simulink library "NCS_Library"  (R2019a)
settings: Solver=VariableStepAuto  StartTime=0.0  StopTime=10.0  RelTol=1e-3
values from neighbouring files (symbols this model uses):
  A = 10    [Parameter.m]
  band = 100000000    [Parameter.m]
  BER = 0    [Parameter.m]
  c = 5000000    [Parameter.m]
  c1 = 4.33    [Parameter.m]
  c2 = 3.16    [Parameter.m]
  CAN2EthernetDelay = 0.000    (= 0)    [Parameter.m]
  cR = 1.5*10^-3    (= 0.0015)    [Parameter.m]
  cw = (cwE * 2 + cwM * (nW_ges-2))/nW_ges    (= 0.1475)    [Parameter.m]
  cwE = 0.35    [Parameter.m]
  cwM = 0.08    [Parameter.m]
  Cycle_Controller = 0    [Parameter.m]
  CyclePLC = 24/1000    (= 0.024)    [Parameter.m]
  d = 800000    [Parameter.m]
  Dr = 0.92    [Parameter.m]
  Ethernet2CANDelay = 0.005    [Parameter.m]
  F_konst = 70892    [Parameter.m]
  FA = 100000    [Parameter.m]
  FB_WB_max = 10000    [Parameter.m]
  FBel_an = iG*nG*F_KZmax*nBan*R_mR/(Dr/2)    (= 28197.4297239)    [Parameter.m]
  FBel_frei = iG*nG*F_KZmax*nBfrei*R_mW/(Dr/2)    (= 29270.6882948)    [Parameter.m]
  Fmaxdyn = 300000    [Parameter.m]
  g = 9.81    [Parameter.m]
  i = 0    [Parameter.m]
  J = 1/2*mA*(Dr/2)^2    (= 158.7)    [Parameter.m]
  k1 = 0.095    [Parameter.m]
  k2 = 9.26/3.6    (= 2.57222222222)    [Parameter.m]
  k3 = 4.63/3.6    (= 1.28611111111)    [Parameter.m]
  mges = 58000    [Parameter.m]
  mu = [mu1 mu2]    [Parameter.m]
  muBel1 = 0.42    [Parameter.m]
  muBel2 = 0.36    [Parameter.m]
  n = 0.001    [Parameter.m]
  n_Mg = 4    [Parameter.m]
  n_WB = 4    [Parameter.m]
  nA = 4    [Parameter.m]
  nBan = 2    [Parameter.m]
  nBfrei = 3    [Parameter.m]
  nM = 4    [Parameter.m]
  nW_an = 4    [Parameter.m]
  P_max = 8200000    [Parameter.m]
  Q = 10    [Parameter.m]
  r_reib = 600    [Parameter.m]
  rho = 1.08    [Parameter.m]
  rhoL = 1.225    [Parameter.m]
  Size = 8    [Parameter.m]
  slip = [s1 s2]    [Parameter.m]
  tol = 0.05    [Parameter.m]
  v00 = 100/3.6    (= 27.7777777778)    [Parameter.m]
  v_grenz = 60/3.6    (= 16.6666666667)    [Parameter.m]
  v_opt = 75/3.6    (= 20.8333333333)    [Parameter.m]
  W_opt = 0.5    [Parameter.m]
  WB = 1    [Parameter.m]
  y_opt = sqrt(W_opt)/((1+sqrt(W_opt))^2+W_opt)    [Parameter.m]
undefined symbols (not defined in the file or in its folder): BUSCapacity, CableLength, controlGate, D_dyn, D_mg, EnableBurst, EnableToF, entity, Entity_out, Gate, Gate_4, Gate_5, Gate_ACK, Gate_copy, Gate_RX, getData, gettime, I_dyn, I_mg, m, magnitude, P_dyn, P_mg, ReadAttributes, readdata, ReadData, ReadSize, sigbuilder_block, Timeout, ToB, ToF, v0, v_d, v_soll
libraries: simulink x176, $bdroot x102
(part 4 of 12)

== system NCS_Library/Network/ETB/Controller Interface ==
  Rx : Inport
  U : Inport  Port=2
  Clock : Clock
  Compare To Constant : simulink/Logic and Bit Operations/Compare To Constant  relop=>=  const=ToF  OutDataTypeStr=uint8
  Constant : Constant  Value=EnableToF
  Data Type Conversion : DataTypeConversion  OutDataTypeStr=uint8
  Display1 : Display
  Display2 : Display
  Failure Control : $bdroot/Network/Applications/Failure Control  SystemSampleTime=-1
  Failure Control1 : $bdroot/Network/Applications/Failure Control  SystemSampleTime=-1
  Logical Operator : Logic  AllPortsSameDT=off  OutDataTypeStr=boolean
  Parameter : Subsystem
  Subsystem : Subsystem
  Tx : Outport
  Recorder : Outport  Port=2
  Failed : Outport  Port=3
  Y_M : Outport  Port=4
  wires:
  Rx/1 -> Failure Control1/1
  Subsystem/3(TxToBus) -> Failure Control/1
  U/1 -> Subsystem/1(InFromController)
  Subsystem/1(OutToController) -> Y_M/1
  Failure Control1/1 -> Subsystem/3(RxFromBus)
  Parameter/1(Out1) -> Subsystem/2(Parameter)
  Failure Control/1 -> Tx/1
  Compare To Constant/1 -> Logical Operator/1, Display1/1
  Logical Operator/1 -> Data Type Conversion/1, Display2/1
  Clock/1 -> Compare To Constant/1
  Constant/1 -> Logical Operator/2
  Data Type Conversion/1 -> Failed/1
  Subsystem/2(Recorder) -> Recorder/1

== system NCS_Library/Network/ETB/ED ==
  RxFromBus : Inport
  Signal : Inport  Port=2
  Failure Control Rx : $bdroot/Network/Applications/Failure Control  SystemSampleTime=-1
  Failure Control Tx : $bdroot/Network/Applications/Failure Control  SystemSampleTime=-1
  Protocol Stack : Subsystem
  User Interface : Subsystem
  TxToBus : Outport
  Recorder : Outport  Port=2
  ReceivedData : Outport  Port=3
  wires:
  Protocol Stack/2(Recorder) -> Recorder/1
  Protocol Stack/1(Data) -> ReceivedData/1
  Signal/1 -> Protocol Stack/1(Signal)
  RxFromBus/1 -> Failure Control Rx/1
  Protocol Stack/3(TxToBus) -> Failure Control Tx/1
  Failure Control Rx/1 -> Protocol Stack/3(RxFromBus)
  Failure Control Tx/1 -> TxToBus/1
  User Interface/1(Parameter) -> Protocol Stack/2(Parameter)

== system NCS_Library/Network/ETB/Ethernet_2-port_Switch ==
  note: Address_Memory
  from_S : Inport
  from_N : Inport  Port=2
  Address_Storage Poer_S : DataStoreMemory  DataStoreName=S  ReadBeforeWriteMsg=warning  WriteAfterWriteMsg=warning  WriteAfterReadMsg=warning  InitialValue=zeros(1, addstore)  ShowAdditionalParam=off
  Address_Storage Port_N : DataStoreMemory  DataStoreName=N  ReadBeforeWriteMsg=warning  WriteAfterWriteMsg=warning  WriteAfterReadMsg=warning  InitialValue=zeros(1, addstore)  ShowAdditionalParam=off
  Buffer_Full_ Frame_loss1 : EntityTerminator  InputPortMessageModes=m  NumberEntitiesArrived=on
      settings: OutputPortMap=o0
  Buffer_Full_Frame_loss : EntityTerminator  InputPortMessageModes=m  NumberEntitiesArrived=on
      settings: OutputPortMap=o0
  Buffer_fill Control : Subsystem
  Buffer_fill Control1 : Subsystem
  Determine Port_L/R : Subsystem  TreatAsAtomicUnit=on
  Determine Port_N : Subsystem  TreatAsAtomicUnit=on
  Display{,1..3} (4 alike) : Display
  Entity Input Switch : EntityInputSwitch  InputPortMessageModes=m,m  OutputPortMessageModes=m
  Entity Input Switch1 : EntityInputSwitch  InputPortMessageModes=m,m  OutputPortMessageModes=m
  Entity Output Switch : EntityOutputSwitch  InputPortMessageModes=m  OutputPortMessageModes=m,m,m  NumberOutputPorts=3  SwitchingCriterion=From attribute  SwitchAttributeName=Route
      settings: OutputPortMap=o0,o1,o2
  Entity Output Switch1 : EntityOutputSwitch  InputPortMessageModes=m,m  OutputPortMessageModes=m,m  SwitchingCriterion=From control port  SwitchAttributeName=Attribute1
      settings: InputPortMap=u0,u1
  Entity Output Switch2 : EntityOutputSwitch  InputPortMessageModes=m  OutputPortMessageModes=m,m,m  NumberOutputPorts=3  SwitchingCriterion=From attribute  SwitchAttributeName=Route
      settings: OutputPortMap=o0,o1,o2
  Entity Output Switch3 : EntityOutputSwitch  InputPortMessageModes=m,m  OutputPortMessageModes=m,m  SwitchingCriterion=From control port  SwitchAttributeName=Attribute1
      settings: InputPortMap=u0,u1
  Entity Queue : EntityQueue  InputPortMessageModes=m  OutputPortMessageModes=m
      settings: OutputPortMap=o5
  Entity Queue1 : EntityQueue  InputPortMessageModes=m  OutputPortMessageModes=m
      settings: OutputPortMap=o5
  Entity Replicator : EntityReplicator  InputPortMessageModes=m  OutputPortMessageModes=m,m
  Entity Terminator : EntityTerminator  InputPortMessageModes=m
  Not_for_ here_Terminate : EntityTerminator  InputPortMessageModes=m
  Output Buffer N : EntityQueue  InputPortMessageModes=m  OutputPortMessageModes=n,m  Capacity=floor(buffer_size/(2*1500))  NumberEntitiesInBlock=on
      settings: OutputPortMap=o1,o5
  Output Buffer R/L : EntityQueue  InputPortMessageModes=m  OutputPortMessageModes=n,m  Capacity=floor(buffer_size/(2*1500))  NumberEntitiesInBlock=on
      settings: OutputPortMap=o1,o5
  Output_Time_N : EntityServer  InputPortMessageModes=m  OutputPortMessageModes=n,m  Capacity=1  ServiceTimeSource=Attribute  NumberEntitiesDeparted=on
      settings: OutputPortMap=o0,o9
  Output_Time_R/L : EntityServer  InputPortMessageModes=m  OutputPortMessageModes=n,m  Capacity=1  ServiceTimeSource=Attribute  NumberEntitiesDeparted=on
      settings: OutputPortMap=o0,o9
  Swicth_Logic_R/L : EntityServer  InputPortMessageModes=m  OutputPortMessageModes=m  Capacity=1  ServiceTimeValue=CycleSwitch  EntryAction=[entity.Route, entity.ServiceTime] = gate_s(entity.MACDestination, entity.MACSource, entity.Size);
  Switch_Logic_N : EntityServer  InputPortMessageModes=m  OutputPortMessageModes=m  Capacity=1  ServiceTimeValue=CycleSwitch  EntryAction=[entity.Route, entity.ServiceTime] = gate_n(entity.MACDestination, entity.MACSource, entity.Size);
  Terminate_ broadcast_ frame : EntityTerminator  InputPortMessageModes=m
  to_S : Outport
  to_N : Outport  Port=2
  wires:
  Buffer_Full_Frame_loss/1 -> Display1/1
  Buffer_Full_ Frame_loss1/1 -> Display/1
  Output Buffer N/2 -> Output_Time_N/1
  Entity Output Switch3/1 -> Output Buffer N/1
  Output Buffer N/1 -> Buffer_fill Control1/1(In1)
  Buffer_fill Control1/1(Out1) -> Entity Output Switch3/1
  Entity Output Switch3/2 -> Buffer_Full_ Frame_loss1/1
  Output Buffer R/L/2 -> Output_Time_R/L/1
  Entity Output Switch1/1 -> Output Buffer R/L/1
  Output Buffer R/L/1 -> Buffer_fill Control/1(In1)
  Buffer_fill Control/1(Out1) -> Entity Output Switch1/1
  Entity Output Switch1/2 -> Buffer_Full_Frame_loss/1
  from_N/1 -> Entity Queue/1
  Switch_Logic_N/1 -> Entity Output Switch/1
  Output_Time_N/2 -> to_N/1
  from_S/1 -> Entity Queue1/1
  Output_Time_R/L/2 -> to_S/1
  Swicth_Logic_R/L/1 -> Entity Output Switch2/1
  Entity Input Switch/1 -> Entity Output Switch3/2
  Entity Output Switch2/2 -> Entity Input Switch/1
  Entity Output Switch/1 -> Entity Terminator/1
  Entity Output Switch/2 -> Entity Input Switch1/1
  Entity Output Switch/3 -> Entity Input Switch1/2
  Entity Input Switch1/1 -> Entity Output Switch1/2
  Entity Output Switch2/3 -> Entity Replicator/1
  Entity Output Switch2/1 -> Not_for_ here_Terminate/1
  Entity Replicator/1 -> Entity Input Switch/2
  Entity Replicator/2 -> Terminate_ broadcast_ frame/1
  Output_Time_R/L/1 -> Display2/1
  Output_Time_N/1 -> Display3/1
  Entity Queue1/1 -> Swicth_Logic_R/L/1
  Entity Queue/1 -> Switch_Logic_N/1

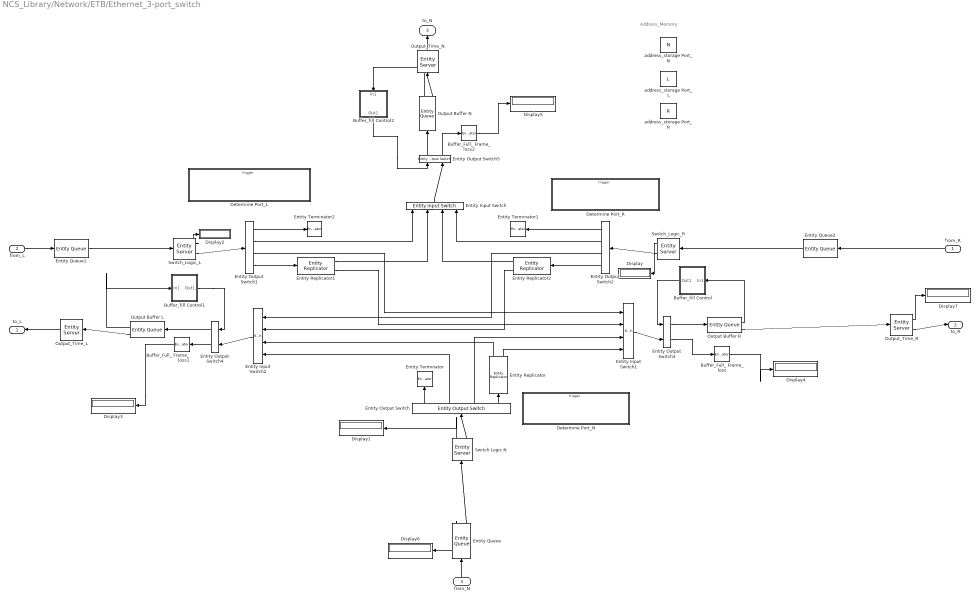
== system NCS_Library/Network/ETB/Ethernet_3-port_switch ==
  note: Address_Memory
  from_R : Inport
  from_L : Inport  Port=2
  from_N : Inport  Port=3
  Buffer_Full_ Frame_loss : EntityTerminator  InputPortMessageModes=m  NumberEntitiesArrived=on
      settings: OutputPortMap=o0
  Buffer_Full_ Frame_loss1 : EntityTerminator  InputPortMessageModes=m  NumberEntitiesArrived=on
      settings: OutputPortMap=o0
  Buffer_Full_ Frame_loss2 : EntityTerminator  InputPortMessageModes=m  NumberEntitiesArrived=on
      settings: OutputPortMap=o0
  Buffer_fill Control : Subsystem
  Buffer_fill Control1 : Subsystem
  Buffer_fill Control2 : Subsystem
  Determine Port_L : Subsystem  TreatAsAtomicUnit=on
  Determine Port_N : Subsystem  TreatAsAtomicUnit=on
  Determine Port_R : Subsystem  TreatAsAtomicUnit=on
  Display{,1..7} (8 alike) : Display
  Entity Input Switch : EntityInputSwitch  InputPortMessageModes=m,m,m,m  OutputPortMessageModes=m  NumberInputPorts=4
      settings: InputPortMap=u1,u2,u3,u4
  Entity Input Switch1 : EntityInputSwitch  InputPortMessageModes=m,m,m,m  OutputPortMessageModes=m  NumberInputPorts=4
      settings: InputPortMap=u1,u2,u3,u4
  Entity Input Switch2 : EntityInputSwitch  InputPortMessageModes=m,m,m,m  OutputPortMessageModes=m  NumberInputPorts=4
      settings: InputPortMap=u1,u2,u3,u4
  Entity Output Switch : EntityOutputSwitch  InputPortMessageModes=m  OutputPortMessageModes=m,m,m,m  NumberOutputPorts=4  SwitchingCriterion=From attribute  SwitchAttributeName=Route
      settings: OutputPortMap=o0,o1,o2,o3
  Entity Output Switch1 : EntityOutputSwitch  InputPortMessageModes=m  OutputPortMessageModes=m,m,m,m  NumberOutputPorts=4  SwitchingCriterion=From attribute  SwitchAttributeName=Route
      settings: OutputPortMap=o0,o1,o2,o3
  Entity Output Switch2 : EntityOutputSwitch  InputPortMessageModes=m  OutputPortMessageModes=m,m,m,m  NumberOutputPorts=4  SwitchingCriterion=From attribute  SwitchAttributeName=Route
      settings: OutputPortMap=o0,o1,o2,o3
  Entity Output Switch3 : EntityOutputSwitch  InputPortMessageModes=m,m  OutputPortMessageModes=m,m  SwitchingCriterion=From control port  SwitchAttributeName=Attribute1
      settings: InputPortMap=u0,u1
  Entity Output Switch4 : EntityOutputSwitch  InputPortMessageModes=m,m  OutputPortMessageModes=m,m  SwitchingCriterion=From control port  SwitchAttributeName=Attribute1
      settings: InputPortMap=u0,u1
  Entity Output Switch5 : EntityOutputSwitch  InputPortMessageModes=m,m  OutputPortMessageModes=m,m  SwitchingCriterion=From control port  SwitchAttributeName=Attribute1
      settings: InputPortMap=u0,u1
  Entity Queue : EntityQueue  InputPortMessageModes=m  OutputPortMessageModes=n,m  NumberEntitiesInBlock=on
      settings: OutputPortMap=o1,o5
  Entity Queue1 : EntityQueue  InputPortMessageModes=m  OutputPortMessageModes=m
      settings: OutputPortMap=o5
  Entity Queue2 : EntityQueue  InputPortMessageModes=m  OutputPortMessageModes=m
      settings: OutputPortMap=o5
  Entity Replicator : EntityReplicator  InputPortMessageModes=m  OutputPortMessageModes=m,m
  Entity Replicator1 : EntityReplicator  InputPortMessageModes=m  OutputPortMessageModes=m,m
  Entity Replicator2 : EntityReplicator  InputPortMessageModes=m  OutputPortMessageModes=m,m
  Entity Terminator : EntityTerminator  InputPortMessageModes=m
  Entity Terminator1 : EntityTerminator  InputPortMessageModes=m
  Entity Terminator2 : EntityTerminator  InputPortMessageModes=m
  Output Buffer L : EntityQueue  InputPortMessageModes=m  OutputPortMessageModes=n,m  Capacity=floor(buffer_size/(3*1500))  NumberEntitiesInBlock=on
      settings: OutputPortMap=o1,o5
  Output Buffer N : EntityQueue  InputPortMessageModes=m  OutputPortMessageModes=n,m  Capacity=floor(buffer_size/(3*1500))  NumberEntitiesInBlock=on
      settings: OutputPortMap=o1,o5
  Output Buffer R : EntityQueue  InputPortMessageModes=m  OutputPortMessageModes=n,m  Capacity=floor(buffer_size/(3*1500))  NumberEntitiesInBlock=on
      settings: OutputPortMap=o1,o5
  Output_Time_L : EntityServer  InputPortMessageModes=m  OutputPortMessageModes=m  Capacity=1  ServiceTimeSource=Attribute
  Output_Time_N : EntityServer  InputPortMessageModes=m  OutputPortMessageModes=m  Capacity=1  ServiceTimeSource=Attribute
  Output_Time_R : EntityServer  InputPortMessageModes=m  OutputPortMessageModes=n,m  Capacity=1  ServiceTimeSource=Attribute  AverageWait=on
      settings: OutputPortMap=o4,o9
  Switch Logic N : EntityServer  InputPortMessageModes=m  OutputPortMessageModes=n,m  Capacity=1  ServiceTimeValue=CycleSwitch  EntryAction=[entity.Route, entity.ServiceTime] = gate_n(entity.MACDestination, entity.MACSource, entity.Size);  NumberEntitiesDeparted=on
      settings: OutputPortMap=o0,o9
  Switch_Logic_L : EntityServer  InputPortMessageModes=m  OutputPortMessageModes=n,m  Capacity=1  ServiceTimeValue=CycleSwitch  EntryAction=[entity.Route, entity.ServiceTime] = gate_l(entity.MACDestination, entity.MACSource, entity.Size);  NumberEntitiesDeparted=on
      settings: OutputPortMap=o0,o9
  Switch_Logic_R : EntityServer  InputPortMessageModes=m  OutputPortMessageModes=n,m  Capacity=1  ServiceTimeValue=CycleSwitch  EntryAction=[entity.Route, entity.ServiceTime] = gate_r(entity.MACDestination, entity.MACSource, entity.Size);  NumberEntitiesDeparted=on
      settings: OutputPortMap=o0,o9
  address_storage Port_L : DataStoreMemory  DataStoreName=L  InitialValue=zeros(1, addstore)  ShowAdditionalParam=off
  address_storage Port_N : DataStoreMemory  DataStoreName=N  InitialValue=zeros(1, addstore)  ShowAdditionalParam=off
  address_storage Port_R : DataStoreMemory  DataStoreName=R  ReadBeforeWriteMsg=warning  WriteAfterWriteMsg=warning  WriteAfterReadMsg=warning  InitialValue=zeros(1, addstore)  ShowAdditionalParam=off
  to_L : Outport
  to_R : Outport  Port=2
  to_N : Outport  Port=3
  wires:
  from_N/1 -> Entity Queue/1
  Switch Logic N/2 -> Entity Output Switch/1
  from_L/1 -> Entity Queue1/1
  Switch_Logic_L/2 -> Entity Output Switch1/1
  Switch_Logic_R/2 -> Entity Output Switch2/1
  from_R/1 -> Entity Queue2/1
  Switch Logic N/1 -> Display1/1
  Output_Time_R/2 -> to_R/1
  Entity Input Switch2/1 -> Entity Output Switch4/2
  Output_Time_L/1 -> to_L/1
  Switch_Logic_L/1 -> Display2/1
  Switch_Logic_R/1 -> Display/1
  Output_Time_R/1 -> Display7/1
  Output Buffer R/2 -> Output_Time_R/1
  Entity Output Switch3/2 -> Buffer_Full_ Frame_loss/1
  Buffer_fill Control/1(Out1) -> Entity Output Switch3/1
  Output Buffer R/1 -> Buffer_fill Control/1(In1)
  Entity Output Switch3/1 -> Output Buffer R/1
  Entity Input Switch1/1 -> Entity Output Switch3/2
  Entity Replicator2/2 -> Entity Input Switch2/2
  Entity Output Switch2/3 -> Entity Input Switch2/1
  Entity Output Switch4/1 -> Output Buffer L/1
  Output Buffer L/1 -> Buffer_fill Control1/1(In1)
  Entity Output Switch4/2 -> Buffer_Full_ Frame_loss1/1
  Buffer_fill Control1/1(Out1) -> Entity Output Switch4/1
  Output Buffer L/2 -> Output_Time_L/1
  Entity Replicator1/2 -> Entity Input Switch1/2
  Entity Output Switch1/2 -> Entity Input Switch/1
  Output_Time_N/1 -> to_N/1
  Entity Output Switch5/1 -> Output Buffer N/1
  Entity Input Switch/1 -> Entity Output Switch5/2
  Output Buffer N/1 -> Buffer_fill Control2/1(In1)
  Entity Output Switch5/2 -> Buffer_Full_ Frame_loss2/1
  Buffer_fill Control2/1(Out1) -> Entity Output Switch5/1
  Output Buffer N/2 -> Output_Time_N/1
  Buffer_Full_ Frame_loss1/1 -> Display3/1
  Buffer_Full_ Frame_loss2/1 -> Display5/1
  Buffer_Full_ Frame_loss/1 -> Display4/1
  Entity Output Switch/1 -> Entity Terminator/1
  Entity Output Switch/2 -> Entity Input Switch2/4
  Entity Output Switch/3 -> Entity Input Switch1/3
  Entity Output Switch/4 -> Entity Replicator/1
  Entity Replicator/2 -> Entity Input Switch1/4
  Entity Replicator/1 -> Entity Input Switch2/3
  Entity Output Switch2/4 -> Entity Replicator2/1
  Entity Output Switch2/1 -> Entity Terminator1/1
  Entity Output Switch2/2 -> Entity Input Switch/4
  Entity Replicator2/1 -> Entity Input Switch/3
  Entity Output Switch1/4 -> Entity Replicator1/1
  Entity Replicator1/1 -> Entity Input Switch/2
  Entity Output Switch1/3 -> Entity Input Switch1/1
  Entity Output Switch1/1 -> Entity Terminator2/1
  Entity Queue2/1 -> Switch_Logic_R/1
  Entity Queue/2 -> Switch Logic N/1
  Entity Queue1/1 -> Switch_Logic_L/1
  Entity Queue/1 -> Display6/1

== system NCS_Library/Network/ETB/OSI Layers ==
  note: Application
  note: Layer 6
  note: Layer 5
  note: Layer 4
  note: Layer 3
  note: Layer 1&2
  Application : Subsystem  mask{Port=1}
      mask Display: disp('App')
  IP : Subsystem
  MAC Controller : Subsystem
  SDTv2 : Subsystem
  TRDP PD : Subsystem
  TRDP Timeout : Subsystem
  UDP Multi-Port : Subsystem
  UDP Single-Port : Subsystem

== system NCS_Library/Network/ETB/Subsystem2 ==
  InSubnet1 : Inport
  InSubnet2 : Inport  Port=2
  InSubnet3 : Inport  Port=3
  MAC Layer : Subsystem
  Routing Layer : Subsystem
  Routing Table : Subsystem
  User Interface : Subsystem
  OutSubnet1 : Outport
  OutSubnet2 : Outport  Port=2
  OutSubnet3 : Outport  Port=3
  wires:
  MAC Layer/3(OutToIP3) -> Routing Layer/4(InSubnet3)
  Routing Layer/1(OutSubnet3) -> MAC Layer/3(InFromIP3)
  MAC Layer/6(OutToSubnet3) -> OutSubnet3/1
  InSubnet3/1 -> MAC Layer/7(InFromSubnet3)
  Routing Table/1(RT) -> Routing Layer/2(Routing Table)
  MAC Layer/5(OutSubnet2) -> OutSubnet2/1
  MAC Layer/4(OutToSubnet1) -> OutSubnet1/1
  InSubnet2/1 -> MAC Layer/6(InFromSubnet2)
  InSubnet1/1 -> MAC Layer/5(InFromSubnet1)
  MAC Layer/2(OutToIP2) -> Routing Layer/5(InSubnet2)
  MAC Layer/1(OutIP1) -> Routing Layer/6(InSubnet1)
  Routing Layer/2(OutSubnet2) -> MAC Layer/2(InFromIP2)
  Routing Layer/3(OutSubnet1) -> MAC Layer/1(InIP1)
  Routing Table/2(FIN) -> Routing Layer/1(FIN)
  User Interface/1(Paramter) -> Routing Table/1(Parameter), Routing Layer/3(Parameter), MAC Layer/4(Parameter)

== system NCS_Library/Network/ETB/Termination ==
  IN : Inport
  Display : Display
  Entity Generator1 : EntityGenerator  InputPortMessageModes=m  OutputPortMessageModes=m  GenerationMethod=Event-based  TimeSource=Signal port  GenerateEntityAtSimulationStart=off  EntityType=Bus object  EntityTypeName=Ethernet_Entity
      settings: InputPortMap=u0
  Entity Terminator : EntityTerminator  InputPortMessageModes=m  NumberEntitiesArrived=on
      settings: OutputPortMap=o0
  Ground1 : Ground
  OUT : Outport
  wires:
  IN/1 -> Entity Terminator/1
  Entity Terminator/1 -> Display/1
  Entity Generator1/1 -> OUT/1
  Ground1/1 -> Entity Generator1/1

== system NCS_Library/Network/Gateway/Gateway1 ==
  In1 : Inport
  CAN Interface : Subsystem
  Ethernet Interface : Subsystem
  Out1 : Outport
  wires:
  CAN Interface/1(OutEthernetData) -> Ethernet Interface/2(CANData)
  Ethernet Interface/2(ReceivedData) -> CAN Interface/1(ReceivedData)
  In1/1 -> Ethernet Interface/1(RxFromBus)
  Ethernet Interface/1(TxToBus) -> Out1/1

== system NCS_Library/Network/Gateway/Gateway2 ==
  In1 : Inport
  CAN Interface : Subsystem
  Ethernet Interface : Subsystem
  Out1 : Outport
  wires:
  Ethernet Interface/1(TxToBus) -> Out1/1
  In1/1 -> Ethernet Interface/1(RxFromBus)
  Ethernet Interface/2(ReceivedData) -> CAN Interface/1(ReceivedData)
  CAN Interface/1(OutEthernetData) -> Ethernet Interface/2(CANData)

== system NCS_Library/Plant (Train)/Angetriebene_Achse/Bremskraft pro angetriebener Achse2 ==
  v : Inport
  f_St,dyn : Inport  Port=2
  f_St_pneumatic : Inport  Port=3
  Add : Sum
  Belagreibwert_Nennwerte : Subsystem
  Belagskraft pro Achse : Constant  Value=FBel_an
  Compare To Constant3 : simulink/Logic and Bit Operations/Compare To Constant  relop=>=  const=0  OutDataTypeStr=boolean
  Display : Display
  Display1 : Display
  Display2 : Display
  Product : Product  Inputs=3
  Product1 : Product  Inputs=3
  Switch : Switch  Criteria=u2 > Threshold
  f_St,dyn1 : InportShadow  Port=2
  max dynamische Bremse pro angetriebener Achse1 : Subsystem
  max dynamische Motor pro angetriebener Achse : Subsystem
  F_B,A : Outport
  wires:
  Belagreibwert_Nennwerte/1(mu_Bel) -> Product/1
  Belagskraft pro Achse/1 -> Product/2
  f_St_pneumatic/1 -> Product/3  "f_St_pneumatic"
  v/1 -> Belagreibwert_Nennwerte/1(v), max dynamische Motor pro angetriebener Achse/1(v), max dynamische Bremse pro angetriebener Achse1/1(v), Compare To Constant3/1
  Product/1 -> Display1/1, Add/2
  Add/1 -> Display2/1, F_B,A/1
  Product1/1 -> Display/1, Add/1
  max dynamische Motor pro angetriebener Achse/1(F_B,dyn_max) -> Switch/3
  Compare To Constant3/1 -> Product1/3
  f_St,dyn/1 -> Product1/1
  max dynamische Bremse pro angetriebener Achse1/1(F_B,dyn_max) -> Switch/1
  f_St,dyn1/1 -> Switch/2
  Switch/1 -> Product1/2

== system NCS_Library/Plant (Train)/Freie_Achse/Bremskraft pro freier Achse1 ==
  v : Inport
  fSt Achse 1 : Inport  Port=2
  Belagreibwert_Nennwerte : Subsystem
  Belagskraft : Constant  Value=FBel_frei
  Display : Display
  Product : Product  Inputs=3
  F_B : Outport
  wires:
  Product/1 -> F_B/1
  Belagreibwert_Nennwerte/1(muBel) -> Product/1
  v/1 -> Belagreibwert_Nennwerte/1(v)
  fSt Achse 1/1 -> Display/1, Product/3
  Belagskraft/1 -> Product/2

== system NCS_Library/Plant (Train)/Kupplung/Dämpferkraft1-2 ==
  v1 : Inport
  v2 : Inport  Port=2
  Add : Sum  Inputs=+-
  Dämpferkonstante : Gain  Gain=d
  Fd1-2 : Outport
  wires:
  Dämpferkonstante/1 -> Fd1-2/1
  Add/1 -> Dämpferkonstante/1
  v2/1 -> Add/2
  v1/1 -> Add/1

== system NCS_Library/Plant (Train)/Kupplung/Federkraft1-2 ==
  s1 : Inport
  s2 : Inport  Port=2
  Add : Sum  Inputs=+-
  Federkonstante : Gain  Gain=c
  Ff1-2 : Outport
  wires:
  Federkonstante/1 -> Ff1-2/1
  Add/1 -> Federkonstante/1
  s2/1 -> Add/2
  s1/1 -> Add/1

== system NCS_Library/Plant (Train)/angetriebener Endwagen Merz/Achse_1 ==
  fSt_dyn : Inport
  fSt Achse 1 : Inport  Port=2
  Wagengeschwindigkeit : Inport  Port=3
  1/I : Gain  Gain=1/J  SaturateOnIntegerOverflow=on  OutDataTypeStr=Inherit: Same as input  ParamDataTypeStr=Inherit: Same as input
  Antriebs-/ Bremsmoment : Scope
  Bremskraft pro angetriebener Achse1 : Subsystem
  Bus Creator : BusCreator  Inputs=3
  Gain : Gain  Gain=1/1000
  Gain1 : Gain  Gain=1/(Dr/2)  SaturateOnIntegerOverflow=on  OutDataTypeStr=Inherit: Same as input  ParamDataTypeStr=Inherit: Same as input
  Kraftschlussbeiwert : Scope
  Max : MinMax  Function=max  Inputs=2
  Neigung : Constant  Value=i
  Product : Product  Inputs=3
  Rad- geschwindigkeit : Integrator  InitialCondition=v0/(Dr/2)  LimitOutput=on  UpperSaturationLimit=1000  LowerSaturationLimit=0
  Radgeschwindigkeit : Scope
  Radradius : Gain  Gain=Dr/2  SaturateOnIntegerOverflow=on  OutDataTypeStr=Inherit: Same as input  ParamDataTypeStr=Inherit: Same as input
  Radradius1 : Gain  Gain=Dr/2  SaturateOnIntegerOverflow=on  OutDataTypeStr=Inherit: Same as input  ParamDataTypeStr=Inherit: Same as input
  Radradius2 : Gain  Gain=Dr/2  SaturateOnIntegerOverflow=on  OutDataTypeStr=Inherit: Same as input  ParamDataTypeStr=Inherit: Same as input
  Schlupf : Fcn  Expr=abs(u(2)-u(1))/u(3)
  Schlupf-Kraftschluss- Beziehung : Lookup_n-D  NumberOfTableDimensions=1  BreakpointsForDimension1=slip  Table=mu  RndMeth=Simplest  SaturateOnIntegerOverflow=on  InputSameDT=on
  Schlupfdiagramm : Scope
  Sign : Signum
  Subtract : Sum  Inputs=-+
  Sum1 : Sum  Inputs=--  SaturateOnIntegerOverflow=on  InputSameDT=on  OutDataTypeStr=Inherit: Same as first input
  Sum2 : Sum  Inputs=+-  SaturateOnIntegerOverflow=on  InputSameDT=on  OutDataTypeStr=Inherit: Same as first input
  Trigonometric Function : Trigonometry  Operator=atan
  Trigonometric Function1 : Trigonometry  Operator=cos
  Weight : Gain  Gain=(mges/4)*g  SaturateOnIntegerOverflow=on  OutDataTypeStr=Inherit: Same as input  ParamDataTypeStr=Inherit: Same as input
  cR : Constant  Value=cR
  Tangentialkraft_A1 : Outport
  wires:
  Gain1/1 -> Bus Creator/2, Max/2, Subtract/2
  fSt Achse 1/1 -> Bremskraft pro angetriebener Achse1/3(Bremsstufenfaktor A1)
  Schlupf/1 -> Schlupf-Kraftschluss- Beziehung/1, Schlupfdiagramm/1
  Sign/1 -> Product/3
  Subtract/1 -> Sign/1
  Max/1 -> Bus Creator/3
  Radradius1/1 -> Bremskraft pro angetriebener Achse1/1(v)
  Product/1 -> Tangentialkraft_A1/1, Radradius2/1
  Bus Creator/1 -> Schlupf/1
  Schlupf-Kraftschluss- Beziehung/1 -> Kraftschlussbeiwert/1, Sum2/2
  Radradius2/1 -> Sum1/2
  Bremskraft pro angetriebener Achse1/1(FBA) -> Radradius/1
  Rad- geschwindigkeit/1 -> Radradius1/1, Radgeschwindigkeit/1, Bus Creator/1, Max/1, Subtract/1
  Radradius/1 -> Sum1/1, Antriebs-/ Bremsmoment/1
  1/I/1 -> Rad- geschwindigkeit/1
  Sum1/1 -> 1/I/1
  Wagengeschwindigkeit/1 -> Gain1/1
  fSt_dyn/1 -> Bremskraft pro angetriebener Achse1/2(fSt_dyn)
  cR/1 -> Sum2/1
  Sum2/1 -> Weight/1
  Neigung/1 -> Gain/1
  Trigonometric Function/1 -> Trigonometric Function1/1
  Gain/1 -> Trigonometric Function/1
  Weight/1 -> Product/2
  Trigonometric Function1/1 -> Product/1

== system NCS_Library/Plant (Train)/angetriebener Endwagen Merz/Achse_2 ==
  fSt_dyn : Inport
  fSt Achse 2 : Inport  Port=2
  Wagengeschwindigkeit : Inport  Port=3
  1/I : Gain  Gain=1/J  SaturateOnIntegerOverflow=on  OutDataTypeStr=Inherit: Same as input  ParamDataTypeStr=Inherit: Same as input
  Bremskraft pro angetriebener Achse2 : Subsystem
  Bus Creator : BusCreator  Inputs=3
  Gain : Gain  Gain=1/1000
  Gain1 : Gain  Gain=1/(Dr/2)  SaturateOnIntegerOverflow=on  OutDataTypeStr=Inherit: Same as input  ParamDataTypeStr=Inherit: Same as input
  Max : MinMax  Function=max  Inputs=2
  Neigung : Constant  Value=i
  Product : Product  Inputs=3
  Rad- geschwindigkeit : Integrator  InitialCondition=v0/(Dr/2)  LimitOutput=on  UpperSaturationLimit=1000  LowerSaturationLimit=0
  Radradius : Gain  Gain=Dr/2  SaturateOnIntegerOverflow=on  OutDataTypeStr=Inherit: Same as input  ParamDataTypeStr=Inherit: Same as input
  Radradius1 : Gain  Gain=Dr/2  SaturateOnIntegerOverflow=on  OutDataTypeStr=Inherit: Same as input  ParamDataTypeStr=Inherit: Same as input
  Radradius2 : Gain  Gain=Dr/2  SaturateOnIntegerOverflow=on  OutDataTypeStr=Inherit: Same as input  ParamDataTypeStr=Inherit: Same as input
  Schlupf : Fcn  Expr=abs(u(2)-u(1))/u(3)
  Schlupf-Kraftschluss- Beziehung : Lookup_n-D  NumberOfTableDimensions=1  BreakpointsForDimension1=slip  Table=mu  RndMeth=Simplest  SaturateOnIntegerOverflow=on  InputSameDT=on
  Sign : Signum
  Subtract : Sum  Inputs=-+
  Sum1 : Sum  Inputs=--  SaturateOnIntegerOverflow=on  InputSameDT=on  OutDataTypeStr=Inherit: Same as first input
  Sum2 : Sum  Inputs=+-  SaturateOnIntegerOverflow=on  InputSameDT=on  OutDataTypeStr=Inherit: Same as first input
  Trigonometric Function : Trigonometry  Operator=atan
  Trigonometric Function1 : Trigonometry  Operator=cos
  Weight : Gain  Gain=(mges/4)*g  SaturateOnIntegerOverflow=on  OutDataTypeStr=Inherit: Same as input  ParamDataTypeStr=Inherit: Same as input
  cR : Constant  Value=cR
  Tangentialkraft_A2 : Outport
  wires:
  Gain1/1 -> Bus Creator/2, Max/2, Subtract/2
  Schlupf/1 -> Schlupf-Kraftschluss- Beziehung/1
  Sign/1 -> Product/3
  Subtract/1 -> Sign/1
  Rad- geschwindigkeit/1 -> Radradius1/1, Max/1, Bus Creator/1, Subtract/1
  Wagengeschwindigkeit/1 -> Gain1/1
  Max/1 -> Bus Creator/3
  Radradius1/1 -> Bremskraft pro angetriebener Achse2/1(v)
  Product/1 -> Tangentialkraft_A2/1, Radradius2/1
  Bus Creator/1 -> Schlupf/1
  Schlupf-Kraftschluss- Beziehung/1 -> Sum2/2
  Radradius2/1 -> Sum1/2
  Bremskraft pro angetriebener Achse2/1(FBA) -> Radradius/1
  Radradius/1 -> Sum1/1
  1/I/1 -> Rad- geschwindigkeit/1
  Sum1/1 -> 1/I/1
  fSt Achse 2/1 -> Bremskraft pro angetriebener Achse2/3(Bremsstufenfaktor A2)
  fSt_dyn/1 -> Bremskraft pro angetriebener Achse2/2(fSt_dyn)
  cR/1 -> Sum2/1
  Sum2/1 -> Weight/1
  Neigung/1 -> Gain/1
  Trigonometric Function/1 -> Trigonometric Function1/1
  Gain/1 -> Trigonometric Function/1
  Weight/1 -> Product/2
  Trigonometric Function1/1 -> Product/1

== system NCS_Library/Plant (Train)/angetriebener Endwagen Merz/Achse_3 ==
  fSt_dyn : Inport
  fSt Achse 3 : Inport  Port=2
  Wagengeschwindigkeit : Inport  Port=3
  1/I : Gain  Gain=1/J  SaturateOnIntegerOverflow=on  OutDataTypeStr=Inherit: Same as input  ParamDataTypeStr=Inherit: Same as input
  Bremskraft pro angetriebener Achse3 : Subsystem
  Bus Creator : BusCreator  Inputs=3
  Gain : Gain  Gain=1/1000
  Gain1 : Gain  Gain=1/(Dr/2)  SaturateOnIntegerOverflow=on  OutDataTypeStr=Inherit: Same as input  ParamDataTypeStr=Inherit: Same as input
  MinMax : MinMax  Function=max  Inputs=2
  Neigung : Constant  Value=i
  Product : Product  Inputs=3
  Rad- geschwindigkeit : Integrator  InitialCondition=v0/(Dr/2)  LimitOutput=on  UpperSaturationLimit=1000  LowerSaturationLimit=0
  Radradius : Gain  Gain=Dr/2  SaturateOnIntegerOverflow=on  OutDataTypeStr=Inherit: Same as input  ParamDataTypeStr=Inherit: Same as input
  Radradius1 : Gain  Gain=Dr/2  SaturateOnIntegerOverflow=on  OutDataTypeStr=Inherit: Same as input  ParamDataTypeStr=Inherit: Same as input
  Radradius2 : Gain  Gain=Dr/2  SaturateOnIntegerOverflow=on  OutDataTypeStr=Inherit: Same as input  ParamDataTypeStr=Inherit: Same as input
  Schlupf : Fcn  Expr=abs(u(2)-u(1))/u(3)
  Schlupf-Kraftschluss- Beziehung : Lookup_n-D  NumberOfTableDimensions=1  BreakpointsForDimension1=slip  Table=mu  RndMeth=Simplest  SaturateOnIntegerOverflow=on  InputSameDT=on
  Sign : Signum
  Subtract : Sum  Inputs=-+
  Sum1 : Sum  Inputs=--  SaturateOnIntegerOverflow=on  InputSameDT=on  OutDataTypeStr=Inherit: Same as first input
  Sum2 : Sum  Inputs=+-  SaturateOnIntegerOverflow=on  InputSameDT=on  OutDataTypeStr=Inherit: Same as first input
  Trigonometric Function : Trigonometry  Operator=atan
  Trigonometric Function1 : Trigonometry  Operator=cos
  Weight : Gain  Gain=(mges/4)*g  SaturateOnIntegerOverflow=on  OutDataTypeStr=Inherit: Same as input  ParamDataTypeStr=Inherit: Same as input
  cR : Constant  Value=cR
  Tangentialkraft_A3 : Outport
  wires:
  Gain1/1 -> Bus Creator/2, MinMax/2, Subtract/2
  Schlupf/1 -> Schlupf-Kraftschluss- Beziehung/1
  Sign/1 -> Product/3
  Subtract/1 -> Sign/1
  Rad- geschwindigkeit/1 -> Radradius1/1, Bus Creator/1, MinMax/1, Subtract/1
  Wagengeschwindigkeit/1 -> Gain1/1
  MinMax/1 -> Bus Creator/3
  Radradius1/1 -> Bremskraft pro angetriebener Achse3/1(v)
  Product/1 -> Tangentialkraft_A3/1, Radradius2/1
  Bus Creator/1 -> Schlupf/1
  Schlupf-Kraftschluss- Beziehung/1 -> Sum2/2
  Radradius2/1 -> Sum1/2
  Bremskraft pro angetriebener Achse3/1(FBA) -> Radradius/1
  Radradius/1 -> Sum1/1
  1/I/1 -> Rad- geschwindigkeit/1
  Sum1/1 -> 1/I/1
  fSt Achse 3/1 -> Bremskraft pro angetriebener Achse3/3(Bremsstufenfaktor A3)
  fSt_dyn/1 -> Bremskraft pro angetriebener Achse3/2(fSt_dyn)
  cR/1 -> Sum2/1
  Sum2/1 -> Weight/1
  Neigung/1 -> Gain/1
  Trigonometric Function/1 -> Trigonometric Function1/1
  Gain/1 -> Trigonometric Function/1
  Weight/1 -> Product/2
  Trigonometric Function1/1 -> Product/1

== system NCS_Library/Plant (Train)/angetriebener Endwagen Merz/Achse_4 ==
  fSt_dyn : Inport
  fSt Achse 4 : Inport  Port=2
  Wagengeschwindigkeit : Inport  Port=3
  1/I : Gain  Gain=1/J  SaturateOnIntegerOverflow=on  OutDataTypeStr=Inherit: Same as input  ParamDataTypeStr=Inherit: Same as input
  Bremskraft pro angetriebener Achse4 : Subsystem
  Bus Creator : BusCreator  Inputs=3
  Display{,1..4} (5 alike) : Display
  Gain1 : Gain  Gain=1/(Dr/2)  SaturateOnIntegerOverflow=on  OutDataTypeStr=Inherit: Same as input  ParamDataTypeStr=Inherit: Same as input
  MinMax : MinMax  Function=max  Inputs=2
  Neigung : Constant  Value=i
  Product : Product  Inputs=3
  Promille : Gain  Gain=1/1000
  Radradius : Gain  Gain=Dr/2  SaturateOnIntegerOverflow=on  OutDataTypeStr=Inherit: Same as input  ParamDataTypeStr=Inherit: Same as input
  Radradius1 : Gain  Gain=Dr/2  SaturateOnIntegerOverflow=on  OutDataTypeStr=Inherit: Same as input  ParamDataTypeStr=Inherit: Same as input
  Radradius2 : Gain  Gain=Dr/2  SaturateOnIntegerOverflow=on  OutDataTypeStr=Inherit: Same as input  ParamDataTypeStr=Inherit: Same as input
  Schlupf : Fcn  Expr=abs(u(2)-u(1))/u(3)
  Schlupf-Kraftschluss- Beziehung : Lookup_n-D  NumberOfTableDimensions=1  BreakpointsForDimension1=slip  Table=mu  RndMeth=Simplest  SaturateOnIntegerOverflow=on  InputSameDT=on
  Sign : Signum
  Subtract : Sum  Inputs=-+
  Sum1 : Sum  Inputs=--  SaturateOnIntegerOverflow=on  InputSameDT=on  OutDataTypeStr=Inherit: Same as first input
  Sum2 : Sum  Inputs=+-  SaturateOnIntegerOverflow=on  InputSameDT=on  OutDataTypeStr=Inherit: Same as first input
  Trigonometric Function : Trigonometry  Operator=atan
  Trigonometric Function1 : Trigonometry  Operator=cos
  Weight : Gain  Gain=(mges/4)*g  SaturateOnIntegerOverflow=on  OutDataTypeStr=Inherit: Same as input  ParamDataTypeStr=Inherit: Same as input
  Wheel Speed : Integrator  InitialCondition=v0/(Dr/2)  LimitOutput=on  UpperSaturationLimit=1000  LowerSaturationLimit=0
  cR : Constant  Value=cR
  Tangentialkraft_A4 : Outport
  wires:
  Gain1/1 -> Bus Creator/2, MinMax/2, Subtract/2
  Schlupf/1 -> Schlupf-Kraftschluss- Beziehung/1
  Sign/1 -> Display/1, Product/3
  Subtract/1 -> Sign/1
  Wheel Speed/1 -> Radradius1/1, Bus Creator/1, MinMax/1, Subtract/1
  Wagengeschwindigkeit/1 -> Display4/1, Gain1/1
  MinMax/1 -> Bus Creator/3
  Radradius1/1 -> Display3/1, Bremskraft pro angetriebener Achse4/1(v)
  Product/1 -> Tangentialkraft_A4/1, Radradius2/1
  Bus Creator/1 -> Schlupf/1
  Schlupf-Kraftschluss- Beziehung/1 -> Sum2/2
  Radradius2/1 -> Display1/1, Sum1/2
  Bremskraft pro angetriebener Achse4/1(FBA) -> Radradius/1
  Radradius/1 -> Display2/1, Sum1/1
  1/I/1 -> Wheel Speed/1
  Sum1/1 -> 1/I/1
  fSt Achse 4/1 -> Bremskraft pro angetriebener Achse4/3(Bremsstufenfaktor A4)
  fSt_dyn/1 -> Bremskraft pro angetriebener Achse4/2(fSt_dyn)
  cR/1 -> Sum2/1
  Sum2/1 -> Weight/1
  Neigung/1 -> Promille/1
  Trigonometric Function/1 -> Trigonometric Function1/1
  Promille/1 -> Trigonometric Function/1
  Weight/1 -> Product/2
  Trigonometric Function1/1 -> Product/1

== system NCS_Library/Plant (Train)/angetriebener Endwagen Merz/Wagen ==
  mu-abhängige Kraft : Inport
  F_vorne : Inport  Port=2
  F_hinten : Inport  Port=3
  Add : Sum  Inputs=++--
  Divide : Product  Inputs=*/
  Fahrwiderstand_Wagen : Subsystem
  Integrator : Integrator  InitialCondition=v0  LimitOutput=on  LowerSaturationLimit=tol  ShowSaturationPort=on
  Integrator1 : Integrator
  Neigung : Constant  Value=i
  Stop Simulation : Stop
  Wagenmasse : Constant  Value=mges
  rho : Gain  Gain=rho
  v : Outport
  a : Outport  Port=2
  s : Outport  Port=3
  wires:
  rho/1 -> Divide/2
  Add/1 -> Divide/1
  Integrator1/1 -> s/1
  Neigung/1 -> Fahrwiderstand_Wagen/2(Neigung in Promille)
  Wagenmasse/1 -> rho/1, Fahrwiderstand_Wagen/3(mges)
  F_vorne/1 -> Add/2
  Integrator/1 -> Integrator1/1, v/1, Fahrwiderstand_Wagen/1(v)
  Fahrwiderstand_Wagen/1(Fw) -> Add/4
  F_hinten/1 -> Add/3
  Divide/1 -> Integrator/1, a/1
  Integrator/2 -> Stop Simulation/1
  mu-abhängige Kraft/1 -> Add/1

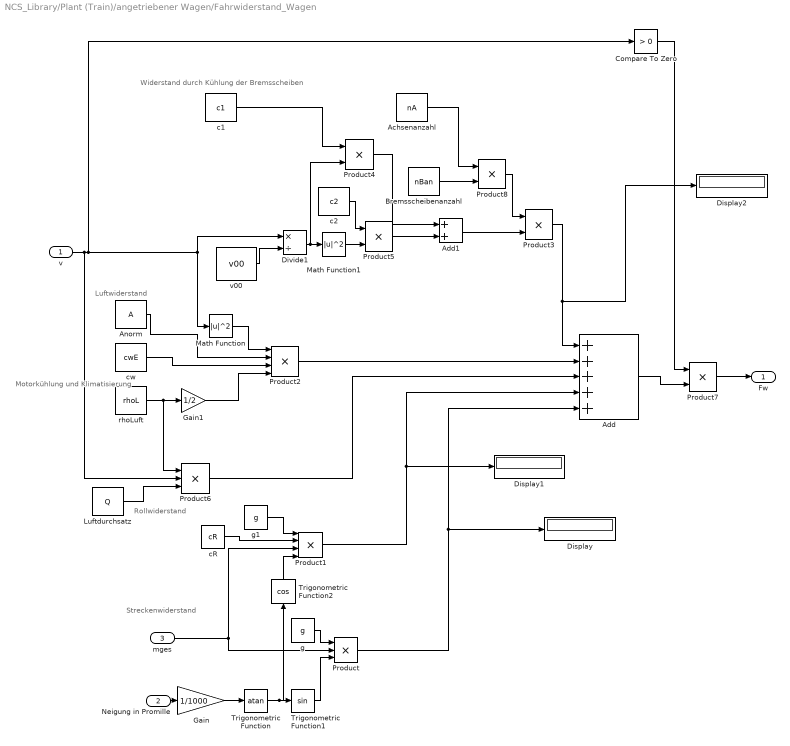
== system NCS_Library/Plant (Train)/angetriebener Wagen/Fahrwiderstand_Wagen ==
  note: Widerstand durch Kühlung der Bremsscheiben
  note: Luftwiderstand
  note: Motorkühlung und Klimatisierung
  note: Rollwiderstand
  note: Streckenwiderstand
  v : Inport
  Neigung in Promille : Inport  Port=2
  mges : Inport  Port=3
  Achsenanzahl : Constant  Value=nA
  Add : Sum  Inputs=+++++
  Add1 : Sum
  Anorm : Constant  Value=A
  Bremsscheibenanzahl : Constant  Value=nBan
  Compare To Zero : simulink/Logic and Bit Operations/Compare To Zero  relop=>  OutDataTypeStr=boolean
  Display : Display
  Display1 : Display
  Display2 : Display
  Divide1 : Product  Inputs=*/
  Gain : Gain  Gain=1/1000
  Gain1 : Gain  Gain=1/2
  Luftdurchsatz : Constant  Value=Q
  Math Function : Math  Operator=magnitude^2  SaturateOnIntegerOverflow=on
  Math Function1 : Math  Operator=magnitude^2  SaturateOnIntegerOverflow=on
  Product : Product  Inputs=3
  Product1 : Product  Inputs=4
  Product2 : Product  Inputs=4
  Product{3..5,7..8} (5 alike) : Product
  Product6 : Product  Inputs=3
  Trigonometric Function : Trigonometry  Operator=atan
  Trigonometric Function1 : Trigonometry
  Trigonometric Function2 : Trigonometry  Operator=cos
  c1 : Constant  Value=c1
  c2 : Constant  Value=c2
  cR : Constant  Value=cR
  cw : Constant  Value=cwE
  g : Constant  Value=g
  g1 : Constant  Value=g
  rhoLuft : Constant  Value=rhoL
  v00 : Constant  Value=v00
  Fw : Outport
  wires:
  Trigonometric Function2/1 -> Product1/4
  Bremsscheibenanzahl/1 -> Product8/2
  Product8/1 -> Product3/1
  Compare To Zero/1 -> Product7/1
  Product7/1 -> Fw/1
  Math Function1/1 -> Product5/2
  Product6/1 -> Add/3
  Luftdurchsatz/1 -> Product6/3
  c2/1 -> Product5/1
  Math Function/1 -> Product2/1
  Divide1/1 -> Math Function1/1, Product4/2
  Product5/1 -> Add1/2
  Product4/1 -> Add1/1
  v00/1 -> Divide1/2
  c1/1 -> Product4/1
  Add1/1 -> Product3/2
  Product3/1 -> Display2/1, Add/1
  Achsenanzahl/1 -> Product8/1
  Product2/1 -> Add/2
  Gain1/1 -> Product2/4
  cw/1 -> Product2/3
  Anorm/1 -> Product2/2
  v/1 -> Math Function/1, Divide1/1, Compare To Zero/1, Product6/2
  rhoLuft/1 -> Gain1/1, Product6/1
  Product1/1 -> Display1/1, Add/4
  mges/1 -> Product1/3, Product/2
  cR/1 -> Product1/2
  g1/1 -> Product1/1
  Add/1 -> Product7/2
  Product/1 -> Add/5, Display/1
  Trigonometric Function1/1 -> Product/3
  g/1 -> Product/1
  Gain/1 -> Trigonometric Function/1
  Trigonometric Function/1 -> Trigonometric Function1/1, Trigonometric Function2/1
  Neigung in Promille/1 -> Gain/1

== system NCS_Library/Plant (Train)/freier Wagen/Bremskraft Schienenbremse ==
  v : Inport
  fSt WB : Inport  Port=2
  Add : Sum
  Compare To Zero : simulink/Logic and Bit Operations/Compare To Zero  relop=>  OutDataTypeStr=boolean
  Constant : Constant  Value=WB
  Display : Display
  Display1 : Display
  Logical Operator : Logic  Operator=NOT  AllPortsSameDT=off  OutDataTypeStr=boolean
  Mg-Bremse pro Wagen : Subsystem
  Product : Product  Inputs=3
  Product1 : Product  Inputs=3
  WB Bremse pro Wagen : Subsystem
  FB_frei : Outport
  wires:
  Product1/1 -> Add/2, Display/1
  Product/1 -> Display1/1, Add/1
  fSt WB/1 -> Product/3, Product1/1
  Mg-Bremse pro Wagen/1(Out1) -> Product/1
  WB Bremse pro Wagen/1(Fb_WB) -> Product1/3
  v/1 -> Mg-Bremse pro Wagen/1(v), WB Bremse pro Wagen/1(v)
  Add/1 -> FB_frei/1
  Constant/1 -> Compare To Zero/1
  Compare To Zero/1 -> Product1/2, Logical Operator/1
  Logical Operator/1 -> Product/2

== system NCS_Library/Plant (Train)/freier Wagen/Fahrwiderstand_Wagen ==
  note: Widerstand durch Kühlung der Bremsscheiben
  note: Luftwiderstand
  note: Motorkühlung und Klimatisierung
  note: Rollwiderstand
  note: Streckenwiderstand
  Neigung in Promille : Inport
  v : Inport  Port=2
  mges : Inport  Port=3
  Achsenanzahl : Constant  Value=nA
  Add : Sum  Inputs=+++++
  Add1 : Sum
  Anorm : Constant  Value=A
  Bremsscheiben : Constant  Value=nBfrei
  Compare To Zero : simulink/Logic and Bit Operations/Compare To Zero  relop=>  OutDataTypeStr=boolean
  Divide1 : Product  Inputs=*/
  Gain : Gain  Gain=1/1000
  Gain1 : Gain  Gain=1/2
  Luftdurchsatz : Constant  Value=Q
  Math Function : Math  Operator=magnitude^2  SaturateOnIntegerOverflow=on
  Math Function1 : Math  Operator=magnitude^2  SaturateOnIntegerOverflow=on
  Product : Product  Inputs=3
  Product1 : Product  Inputs=4
  Product2 : Product  Inputs=4
  Product{3..5,7..8} (5 alike) : Product
  Product6 : Product  Inputs=3
  Trigonometric Function : Trigonometry  Operator=atan
  Trigonometric Function1 : Trigonometry
  Trigonometric Function2 : Trigonometry  Operator=cos
  c1 : Constant  Value=c1
  c2 : Constant  Value=c2
  cR : Constant  Value=cR
  cw : Constant  Value=cwM
  g : Constant  Value=g
  g1 : Constant  Value=g
  rhoLuft : Constant  Value=rhoL
  v00 : Constant  Value=v00
  Fw : Outport
  wires:
  Trigonometric Function2/1 -> Product1/4
  Bremsscheiben/1 -> Product8/2
  Product8/1 -> Product3/1
  Compare To Zero/1 -> Product7/1
  Product7/1 -> Fw/1
  Math Function1/1 -> Product5/2
  Product6/1 -> Add/3
  Luftdurchsatz/1 -> Product6/3
  c2/1 -> Product5/1
  Math Function/1 -> Product2/1
  Divide1/1 -> Math Function1/1, Product4/2
  Product5/1 -> Add1/2
  Product4/1 -> Add1/1
  v00/1 -> Divide1/2
  c1/1 -> Product4/1
  Add1/1 -> Product3/2
  Product3/1 -> Add/1
  Achsenanzahl/1 -> Product8/1
  Product2/1 -> Add/2
  Gain1/1 -> Product2/4
  cw/1 -> Product2/3
  Anorm/1 -> Product2/2
  v/1 -> Math Function/1, Divide1/1, Compare To Zero/1, Product6/2
  rhoLuft/1 -> Gain1/1, Product6/1
  Product1/1 -> Add/4
  mges/1 -> Product1/3, Product/2
  cR/1 -> Product1/2
  g1/1 -> Product1/1
  Add/1 -> Product7/2
  Product/1 -> Add/5
  Trigonometric Function1/1 -> Product/3
  g/1 -> Product/1
  Gain/1 -> Trigonometric Function/1
  Trigonometric Function/1 -> Trigonometric Function1/1, Trigonometric Function2/1
  Neigung in Promille/1 -> Gain/1

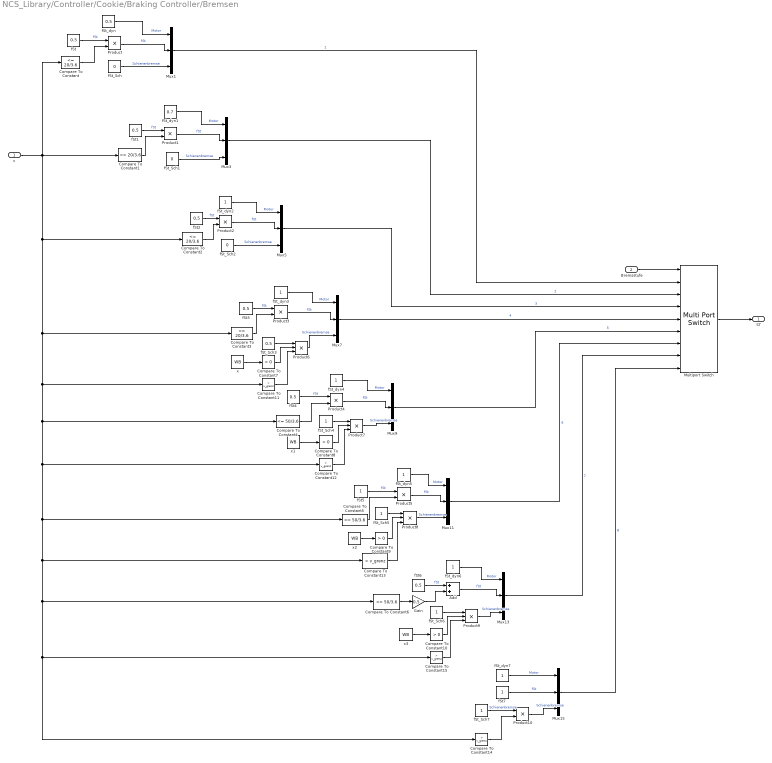
== system NCS_Library/Controller/Cookie/Braking Controller/Bremsen ==
  v : Inport
  Bremsstufe : Inport  Port=2
  Add : Sum
  Compare To Constant{,1..3} (4 alike) : simulink/Logic and Bit Operations/Compare To Constant  relop=<=  const=20/3.6  OutDataTypeStr=boolean
  Compare To Constant{7..10} (4 alike) : simulink/Logic and Bit Operations/Compare To Constant  relop=>  const=0  OutDataTypeStr=boolean
  Compare To Constant{11..15} (5 alike) : simulink/Logic and Bit Operations/Compare To Constant  relop=>  const=v_grenz  OutDataTypeStr=boolean
  Compare To Constant4 : simulink/Logic and Bit Operations/Compare To Constant  relop=<=  const=50/3.6  OutDataTypeStr=boolean
  Compare To Constant5 : simulink/Logic and Bit Operations/Compare To Constant  relop=<=  const=50/3.6  OutDataTypeStr=boolean
  Compare To Constant6 : simulink/Logic and Bit Operations/Compare To Constant  relop=<=  const=50/3.6  OutDataTypeStr=boolean
  Gain : Gain  Gain=0.5
  Multiport Switch : MultiPortSwitch  Inputs=8
  Mux{1,3,5,7,9,11,13,15} (8 alike) : Mux  Inputs=3
  Product{,1..5,10} (7 alike) : Product
  Product{6..9} (4 alike) : Product  Inputs=3
  fSt{,1..4,6} (6 alike) : Constant  Value=0.5
  fSt5 : Constant
  fSt7 : Constant
  fSt_Sch : Constant  Value=0
  fSt_Sch1 : Constant  Value=0
  fSt_Sch2 : Constant  Value=0
  fSt_Sch3 : Constant  Value=0.5
  fSt_Sch{4..7} (4 alike) : Constant
  fSt_dyn : Constant  Value=0.5
  fSt_dyn1 : Constant  Value=0.7
  fSt_dyn{2..7} (6 alike) : Constant
  x{,1..3} (4 alike) : Constant  Value=WB
  ST : Outport
  wires:
  Compare To Constant15/1 -> Product9/3
  Compare To Constant14/1 -> Product10/2
  Product10/1 -> Mux15/3  "Schienenbremse"
  Compare To Constant13/1 -> Product8/3
  Compare To Constant12/1 -> Product7/3
  Compare To Constant11/1 -> Product6/3
  Compare To Constant10/1 -> Product9/2
  x3/1 -> Compare To Constant10/1
  fSt_Sch6/1 -> Product9/1
  Compare To Constant9/1 -> Product8/2
  x2/1 -> Compare To Constant9/1
  fSt_Sch5/1 -> Product8/1
  Compare To Constant8/1 -> Product7/2
  x1/1 -> Compare To Constant8/1
  fSt_Sch4/1 -> Product7/1
  Compare To Constant7/1 -> Product6/2
  x/1 -> Compare To Constant7/1
  fSt_Sch3/1 -> Product6/1
  Gain/1 -> Add/2
  fSt6/1 -> Add/1  "fSt"
  Compare To Constant6/1 -> Gain/1
  fSt5/1 -> Product5/1  "fSt"
  Compare To Constant5/1 -> Product5/2
  fSt4/1 -> Product4/1  "fSt"
  Compare To Constant4/1 -> Product4/2
  fSt3/1 -> Product3/1  "fSt"
  Compare To Constant3/1 -> Product3/2
  fSt2/1 -> Product2/1  "fSt"
  Compare To Constant2/1 -> Product2/2
  Compare To Constant1/1 -> Product1/2
  fSt1/1 -> Product1/1  "fSt"
  v/1 -> Compare To Constant1/1, Compare To Constant/1, Compare To Constant2/1, Compare To Constant3/1, Compare To Constant11/1, Compare To Constant4/1, Compare To Constant12/1, Compare To Constant5/1, Compare To Constant14/1, Compare To Constant15/1, Compare To Constant6/1, Compare To Constant13/1
  Compare To Constant/1 -> Product/2
  fSt/1 -> Product/1  "fSt"
  Bremsstufe/1 -> Multiport Switch/1
  Mux15/1 -> Multiport Switch/9  "8"
  fSt_dyn7/1 -> Mux15/1  "Motor"
  fSt_Sch7/1 -> Product10/1  "Schienenbremse"
  fSt7/1 -> Mux15/2  "fSt"
  Mux13/1 -> Multiport Switch/8  "7"
  fSt_dyn6/1 -> Mux13/1  "Motor"
  Product9/1 -> Mux13/3  "Schienenbremse"
  Add/1 -> Mux13/2  "fSt"
  Mux11/1 -> Multiport Switch/7  "6"
  fSt_dyn5/1 -> Mux11/1  "Motor"
  Product8/1 -> Mux11/3  "Schienenbremse"
  Product5/1 -> Mux11/2  "fSt"
  Mux9/1 -> Multiport Switch/6  "5"
  fSt_dyn4/1 -> Mux9/1  "Motor"
  Product7/1 -> Mux9/3  "Schienenbremse"
  Product4/1 -> Mux9/2  "fSt"
  Mux7/1 -> Multiport Switch/5  "4"
  fSt_dyn3/1 -> Mux7/1  "Motor"
  Product6/1 -> Mux7/3  "Schienenbremse"
  Product3/1 -> Mux7/2  "fSt"
  Mux5/1 -> Multiport Switch/4  "3"
  fSt_dyn2/1 -> Mux5/1  "Motor"
  fSt_Sch2/1 -> Mux5/3  "Schienenbremse"
  Product2/1 -> Mux5/2  "fSt"
  Mux3/1 -> Multiport Switch/3  "2"
  fSt_dyn1/1 -> Mux3/1  "Motor"
  fSt_Sch1/1 -> Mux3/3  "Schienenbremse"
  Product1/1 -> Mux3/2  "fSt"
  Mux1/1 -> Multiport Switch/2  "1"
  fSt_dyn/1 -> Mux1/1  "Motor"
  fSt_Sch/1 -> Mux1/3  "Schienenbremse"
  Product/1 -> Mux1/2  "fSt"
  Multiport Switch/1 -> ST/1

== system NCS_Library/Controller/Cookie/Braking Controller/Leerlauf ==
  F_B : Constant  Value=0
  Mux1 : Mux  Inputs=3
  fSt : Constant  Value=0
  fSt_Sch : Constant  Value=0
  ST : Outport
  wires:
  Mux1/1 -> ST/1
  fSt_Sch/1 -> Mux1/3  "Schienenbremse"
  fSt/1 -> Mux1/2  "fSt"
  F_B/1 -> Mux1/1  "Motor"

== system NCS_Library/Controller/Cookie/Braking Controller/Notbremsung ==
  v : Inport
  Compare To Constant : simulink/Logic and Bit Operations/Compare To Constant  relop=>  const=v_grenz  OutDataTypeStr=boolean
  Mux2 : Mux  Inputs=3
  Product9 : Product
  fSt : Constant
  fSt_Sch : Constant
  fSt_dyn : Constant
  ST : Outport
  wires:
  Compare To Constant/1 -> Product9/2
  v/1 -> Compare To Constant/1
  fSt_Sch/1 -> Product9/1  "Schienenbremse"
  fSt_dyn/1 -> Mux2/1  "fSt_dyn"
  Product9/1 -> Mux2/3  "Schienenbremse"
  fSt/1 -> Mux2/2  "fSt"
  Mux2/1 -> ST/1
